simulink model "Driveline_ctrl_sim"  (R2020a)
settings: Solver=ode45  StartTime=0.0  StopTime=10  MaxStep=0.001  RelTol=1e-3
values from neighbouring files (symbols this model uses):
  A = [[0 1 0 0 0];[-(cw+cs)/mw -ds/mw cs/mw ds/mw -1/mw];[0 0 0 1 0];[cs/mc ds/mc -cs/mc -ds/mc 1/mc];[0 0 0 0 -1/tau]]    [active_suspension_ctrl_design.m]
undefined symbols (not defined in the file or in its folder): Bd, Bu, Cp, d, K, kr, L
settings Model: Creator=jofr  LastModifiedBy=juan
settings DataIOCC: LimitDataPoints=on  SaveFormat=Array  SignalLoggingSaveFormat=ModelDataLogs  ReturnWorkspaceOutputs=off
settings OptimizationCC: BlockReduction=off  BooleanDataType=off  LifeSpan=inf
settings DebuggingCC: SaveWithParameterizedLinksMsg=none  UnderspecifiedInitializationDetection=Classic  MergeDetectMultiDrivingBlocksExec=none  SignalResolutionControl=TryResolveAllWithWarning  MultiTaskDSMMsg=warning  MultiTaskCondExecSysMsg=none  SFUnexpectedBacktrackingDiag=warning  SFNoUnconditionalDefaultTransitionDiag=warning  SFExecutionAtInitializationDiag=none  ArithmeticOperatorsInVariantConditions=warning
settings HardwareCC: ProdBitPerPointer=32  ProdBitPerSizeT=32  ProdBitPerPtrDiffT=32  ProdLargestAtomicFloat=None  ProdIntDivRoundTo=Undefined  ProdEndianess=Unspecified  ProdWordSize=32  ProdHWDeviceType=32-bit Generic  TargetUnknown=on
settings ModelReferenceCC: PropagateSignalLabelsOutOfModel=off
settings SFSimCC: SimUseLocalCustomCode=off  CustomCodeUndefinedFunction=UseInterfaceOnly
settings RTWCC: RTWUseLocalCustomCode=off
settings CodeAppCC: StateflowObjectComments=on
settings GRTTargetCC: TargetLangStandard=C89/C90 (ANSI)
settings ConfigComp: CovMetricSettings=dw  CovHtmlReporting=on  CovSaveCumulativeToWorkspaceVar=on  CovSaveSingleToWorkspaceVar=on  CovExternalEMLEnable=off

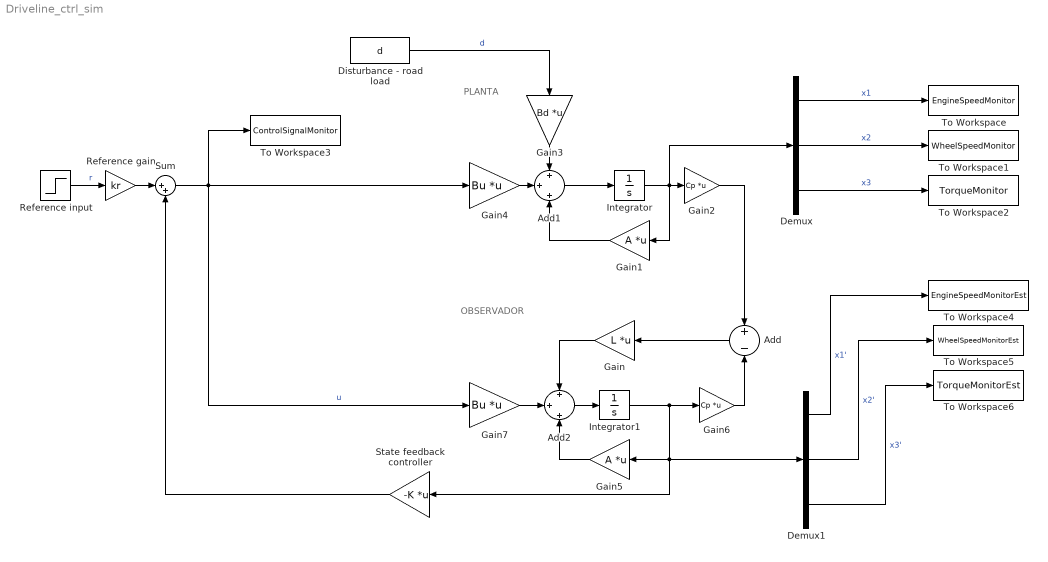
== system Driveline_ctrl_sim ==
  note: OBSERVADOR
  note: PLANTA
  Add : Sum  Inputs=+-
  Add1 : Sum  Inputs=+|+|+
  Add2 : Sum  Inputs=+|+|+
  Demux : Demux  Outputs=3
  Demux1 : Demux  Outputs=3
  Disturbance - road load : Constant  Value=d
  Gain : Gain  Gain=L  Multiplication=Matrix(K*u)
  Gain1 : Gain  Gain=A  Multiplication=Matrix(K*u)
  Gain2 : Gain  Gain=Cp  Multiplication=Matrix(K*u)
  Gain3 : Gain  Gain=Bd  Multiplication=Matrix(K*u)
  Gain4 : Gain  Gain=Bu  Multiplication=Matrix(K*u)
  Gain5 : Gain  Gain=A  Multiplication=Matrix(K*u)
  Gain6 : Gain  Gain=Cp  Multiplication=Matrix(K*u)
  Gain7 : Gain  Gain=Bu  Multiplication=Matrix(K*u)
  Integrator : Integrator
  Integrator1 : Integrator
  Reference gain : Gain  Gain=kr
  Reference input : Step  Before=2  After=4  SampleTime=0
  State feedback controller : Gain  Gain=-K  Multiplication=Matrix(K*u)
  Sum : Sum  Inputs=|++
  To Workspace : ToWorkspace  VariableName=EngineSpeedMonitor  SaveFormat=Structure With Time  SampleTime=-1
  To Workspace1 : ToWorkspace  VariableName=WheelSpeedMonitor  SaveFormat=Structure With Time  SampleTime=-1
  To Workspace2 : ToWorkspace  VariableName=TorqueMonitor  SaveFormat=Structure With Time  SampleTime=-1
  To Workspace3 : ToWorkspace  VariableName=ControlSignalMonitor  SaveFormat=Structure With Time  SampleTime=-1
  To Workspace4 : ToWorkspace  VariableName=EngineSpeedMonitorEst  SaveFormat=Structure With Time  SampleTime=-1
  To Workspace5 : ToWorkspace  VariableName=WheelSpeedMonitorEst  SaveFormat=Structure With Time  SampleTime=-1
  To Workspace6 : ToWorkspace  VariableName=TorqueMonitorEst  SaveFormat=Structure With Time  SampleTime=-1
  wires:
  Demux/1 -> To Workspace/1  "x1"
  State feedback controller/1 -> Sum/2
  Reference input/1 -> Reference gain/1  "r"
  Sum/1 -> Gain4/1, Gain7/1, To Workspace3/1  "u"
  Reference gain/1 -> Sum/1
  Demux/2 -> To Workspace1/1  "x2"
  Demux/3 -> To Workspace2/1  "x3"
  Integrator/1 -> Demux/1, Gain1/1, Gain2/1
  Gain2/1 -> Add/1
  Gain4/1 -> Add1/2
  Add1/1 -> Integrator/1
  Disturbance - road load/1 -> Gain3/1  "d"
  Gain3/1 -> Add1/1
  Gain1/1 -> Add1/3
  Integrator1/1 -> Demux1/1, Gain5/1, State feedback controller/1, Gain6/1
  Gain5/1 -> Add2/3
  Gain7/1 -> Add2/2
  Gain6/1 -> Add/2
  Add2/1 -> Integrator1/1
  Gain/1 -> Add2/1
  Add/1 -> Gain/1
  Demux1/1 -> To Workspace4/1  "x1'"
  Demux1/2 -> To Workspace5/1  "x2'"
  Demux1/3 -> To Workspace6/1  "x3'"
